simulink model "chybadobrze"  (R2022a)
settings: Solver=VariableStepAuto  StartTime=0.0  StopTime=30  RelTol=1e-3
settings Model: Creator=radek  LastModifiedBy=radek

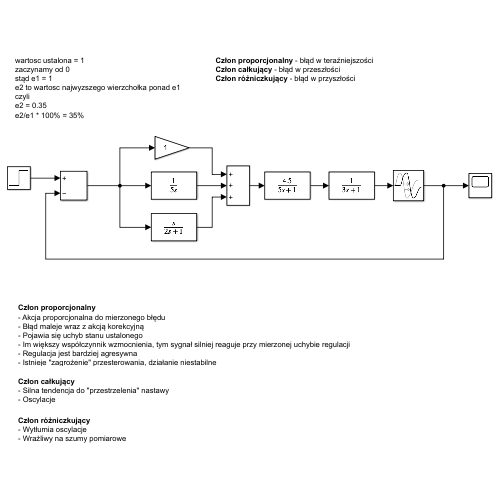
[thumbnail: Simulink's stored preview of the top-level diagram]
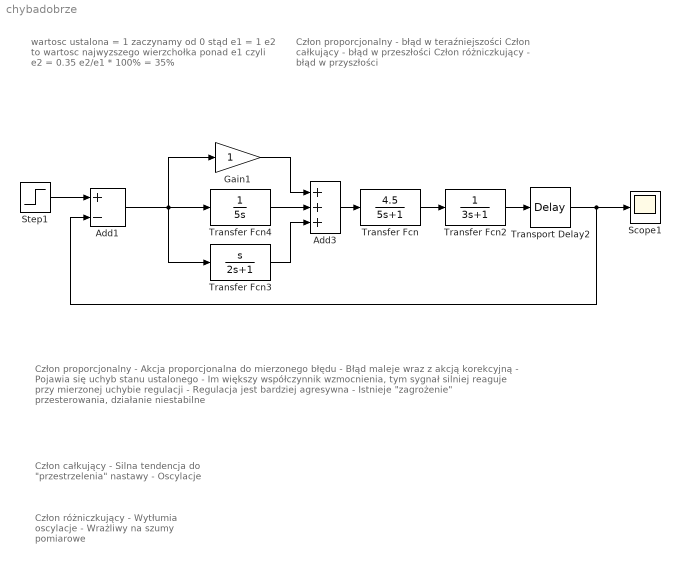
== system chybadobrze ==
  note: Człon różniczkujący
      | - Wytłumia oscylacje
      | - Wrażliwy na szumy pomiarowe
  note: Człon całkujący
      | - Silna tendencja do "przestrzelenia" nastawy
      | - Oscylacje
  note: Człon proporcjonalny
      | - Akcja proporcjonalna do mierzonego błędu
      | - Błąd maleje wraz z akcją korekcyjną
      | - Pojawia się uchyb stanu ustalonego
      | - Im większy współczynnik wzmocnienia, tym sygnał silniej reaguje przy mierzonej uchybie regulacji
      | - Regulacja jest bardziej agresywna
      | - Istnieje "zagrożenie" przesterowania, działanie niestabilne
  note: Człon proporcjonalny - błąd w teraźniejszości
      | Człon całkujący - błąd w przeszłości
      | Człon różniczkujący - błąd w przyszłości
  note: wartosc ustalona = 1
      | zaczynamy od 0
      | stąd e1 = 1
      | e2 to wartosc najwyzszego wierzchołka ponad e1
      | czyli
      | e2 = 0.35
      | e2/e1 * 100% = 35%
  Add1 : Sum  Inputs=+-
  Add3 : Sum  Inputs=+++
  Gain1 : Gain
  Scope1 : Scope
  Step1 : Step  Time=0  SampleTime=0
  Transfer Fcn : TransferFcn  Numerator=[4.5]  Denominator=[5 1]
  Transfer Fcn2 : TransferFcn  Denominator=[3 1]
  Transfer Fcn3 : TransferFcn  Numerator=[1 0]  Denominator=[2 1]
  Transfer Fcn4 : TransferFcn  Denominator=[5 0]
  Transport Delay2 : TransportDelay  DelayTime=exp(-2)
  wires:
  Step1/1 -> Add1/1
  Transport Delay2/1 -> Add1/2, Scope1/1
  Transfer Fcn2/1 -> Transport Delay2/1
  Add3/1 -> Transfer Fcn/1
  Transfer Fcn/1 -> Transfer Fcn2/1
  Gain1/1 -> Add3/1
  Add1/1 -> Gain1/1, Transfer Fcn4/1, Transfer Fcn3/1
  Transfer Fcn3/1 -> Add3/3
  Transfer Fcn4/1 -> Add3/2
